simulink model "gm_HDL_pfc_gold_fi_og_vnl"  (R2024b)
settings: Solver=FixedStepDiscrete  StartTime=0.0  StopTime=.2  RelTol=1e-3
InitFcn:
  | fidelity_pfc_vals;
  | nbits=(2^12)-2;
  | load('C:\Users\Angel\Desktop\hil\pfc3ph\matlab\sim\sschdl\pfc_desktop\stateSpaceParameters.mat');
undefined symbols (not defined in the file or in its folder): a, b, c, DiscIntNeverNeededParam, fsw, Gs, s, stateSpaceParameters_1, t_ss, tsw
libraries: simulink x47, hdlmdlgenlib x24, hdlsllib x10, mcbcontrolslib x5, dspsrcs4 x3, slpidlib x2, hdlssclib x2, spsSVPWMGenerator2LevelLib x1, spsPLL3phLib x1, fillib x1
(part 5 of 5)

== system gm_HDL_pfc_gold_fi_og_vnl/simscape_system/simscape_system/HDL Subsystem/Sparse Matrix-Vector Product3/hNNewMatrixD_shared/Serializer_Subnetwork ==
  in0 : Inport  OutDataTypeStr=fixdt(1, 25, 19)  PortDimensions=[140]  SampleTime=1.38600138600139e-08
  in1 : Inport  Port=2  OutDataTypeStr=fixdt(0, 5, 0)  SampleTime=1.38600138600139e-08
  ratechange_splitcomp : Demux  Outputs=20
  splitcomp_multiport : MultiPortSwitch  DataPortOrder=Zero-based contiguous  Inputs=20  DiagnosticForDefault=None  zeroidx=on  OutDataTypeStr=fixdt(1, 25, 19)  SampleTime=1.38600138600139e-08  SaturateOnIntegerOverflow=off  InputSameDT=off
  out0 : Outport  OutDataTypeStr=fixdt(1, 25, 19)  PortDimensions=[7]  SampleTime=1.38600138600139e-08
  wires:
  splitcomp_multiport/1 -> out0/1
  ratechange_splitcomp/20 -> splitcomp_multiport/21
  ratechange_splitcomp/19 -> splitcomp_multiport/20
  ratechange_splitcomp/14 -> splitcomp_multiport/15
  ratechange_splitcomp/16 -> splitcomp_multiport/17
  ratechange_splitcomp/13 -> splitcomp_multiport/14
  ratechange_splitcomp/15 -> splitcomp_multiport/16
  ratechange_splitcomp/12 -> splitcomp_multiport/13
  ratechange_splitcomp/10 -> splitcomp_multiport/11
  ratechange_splitcomp/17 -> splitcomp_multiport/18
  ratechange_splitcomp/7 -> splitcomp_multiport/8
  ratechange_splitcomp/9 -> splitcomp_multiport/10
  ratechange_splitcomp/6 -> splitcomp_multiport/7
  ratechange_splitcomp/8 -> splitcomp_multiport/9
  ratechange_splitcomp/4 -> splitcomp_multiport/5
  in1/1 -> splitcomp_multiport/1
  ratechange_splitcomp/1 -> splitcomp_multiport/2
  in0/1 -> ratechange_splitcomp/1
  ratechange_splitcomp/2 -> splitcomp_multiport/3
  ratechange_splitcomp/3 -> splitcomp_multiport/4
  ratechange_splitcomp/5 -> splitcomp_multiport/6
  ratechange_splitcomp/11 -> splitcomp_multiport/12
  ratechange_splitcomp/18 -> splitcomp_multiport/19

== system gm_HDL_pfc_gold_fi_og_vnl/simscape_system/simscape_system/HDL Subsystem/Sparse Matrix-Vector Product3/hNNewMatrixD_shared/Serializer_Subnetwork1 ==
  in0 : Inport  OutDataTypeStr=fixdt(1, 25, 13)  PortDimensions=[140]  SampleTime=1.38600138600139e-08
  in1 : Inport  Port=2  OutDataTypeStr=fixdt(0, 5, 0)  SampleTime=1.38600138600139e-08
  ratechange_splitcomp : Demux  Outputs=20
  splitcomp_multiport : MultiPortSwitch  DataPortOrder=Zero-based contiguous  Inputs=20  DiagnosticForDefault=None  zeroidx=on  OutDataTypeStr=fixdt(1, 25, 13)  SampleTime=1.38600138600139e-08  SaturateOnIntegerOverflow=off  InputSameDT=off
  out0 : Outport  OutDataTypeStr=fixdt(1, 25, 13)  PortDimensions=[7]  SampleTime=1.38600138600139e-08
  wires:
  ratechange_splitcomp/16 -> splitcomp_multiport/17
  ratechange_splitcomp/18 -> splitcomp_multiport/19
  ratechange_splitcomp/20 -> splitcomp_multiport/21
  ratechange_splitcomp/14 -> splitcomp_multiport/15
  ratechange_splitcomp/13 -> splitcomp_multiport/14
  ratechange_splitcomp/12 -> splitcomp_multiport/13
  ratechange_splitcomp/11 -> splitcomp_multiport/12
  ratechange_splitcomp/10 -> splitcomp_multiport/11
  ratechange_splitcomp/9 -> splitcomp_multiport/10
  splitcomp_multiport/1 -> out0/1
  ratechange_splitcomp/7 -> splitcomp_multiport/8
  ratechange_splitcomp/3 -> splitcomp_multiport/4
  ratechange_splitcomp/4 -> splitcomp_multiport/5
  ratechange_splitcomp/5 -> splitcomp_multiport/6
  ratechange_splitcomp/1 -> splitcomp_multiport/2
  ratechange_splitcomp/15 -> splitcomp_multiport/16
  ratechange_splitcomp/17 -> splitcomp_multiport/18
  ratechange_splitcomp/19 -> splitcomp_multiport/20
  in1/1 -> splitcomp_multiport/1
  ratechange_splitcomp/2 -> splitcomp_multiport/3
  ratechange_splitcomp/6 -> splitcomp_multiport/7
  ratechange_splitcomp/8 -> splitcomp_multiport/9
  in0/1 -> ratechange_splitcomp/1

== system gm_HDL_pfc_gold_fi_og_vnl/simscape_system/simscape_system/HDL Subsystem/Sparse Matrix-Vector Product3/hNNewMatrixD_shared/counter ==
  globalSchedule : EnablePort  OutDataTypeStr=boolean
  ctr_0_19 : hdlsllib/Sources/HDL Counter  CountType=Count limited  CountInit=double(0)  CountStep=double(1)  CountMax=double(19)  CountFromType=Initial value  CountFrom=double(0)  CountResetPort=off  CountLoadPort=off  CountEnbPort=off  CountDirPort=off  CountHitOutputPort=off  CountDataType=Unsigned  CountWordLen=5  CountFracLen=0  CountSampTime=1.38600138600139e-08
  out0 : Outport  OutDataTypeStr=fixdt(0, 5, 0)  SampleTime=1.38600138600139e-08  InitialOutput=0
  wires:
  ctr_0_19/1 -> out0/1

== system gm_HDL_pfc_gold_fi_og_vnl/simscape_system/simscape_system/HDL Subsystem/Sparse Matrix-Vector Product3/hNNewMatrixD_shared/dot_product1_bypass ==
  in0 : Inport  OutDataTypeStr=fixdt(1, 50, 32)  SampleTime=1.38600138600139e-08
  in1 : Inport  Port=2  OutDataTypeStr=boolean  SampleTime=1.38600138600139e-08
  dot_product1_enb : Switch  Criteria=u2 ~= 0  Threshold=double(0)  OutDataTypeStr=fixdt(1, 50, 32)  SampleTime=1.38600138600139e-08  SaturateOnIntegerOverflow=off  InputSameDT=off
  dot_product1_state : Delay  DelayLength=double(1)  InitialCondition=0  SampleTime=1.38600138600139e-08
  out0 : Outport  OutDataTypeStr=fixdt(1, 50, 32)  SampleTime=1.38600138600139e-08
  wires:
  dot_product1_state/1 -> dot_product1_enb/3
  in1/1 -> dot_product1_enb/2
  in0/1 -> dot_product1_enb/1
  dot_product1_enb/1 -> out0/1, dot_product1_state/1

== system gm_HDL_pfc_gold_fi_og_vnl/simscape_system/simscape_system/HDL Subsystem/Sparse Matrix-Vector Product3/hNNewMatrixD_shared/dot_product_7 ==
  in1 : Inport  OutDataTypeStr=fixdt(1, 25, 19)  PortDimensions=[7]  SampleTime=1.38600138600139e-08
  in2 : Inport  Port=2  OutDataTypeStr=fixdt(1, 25, 13)  PortDimensions=[7]  SampleTime=1.38600138600139e-08
  HwModeRegister : Delay  DelayLength=double(1)  InitialCondition=0  SampleTime=1.38600138600139e-08
  HwModeRegister1 : Delay  DelayLength=double(1)  InitialCondition=0  SampleTime=1.38600138600139e-08
  PipelineRegister : Delay  DelayLength=double(1)  InitialCondition=0  SampleTime=1.38600138600139e-08
  adder{,1..5} (6 alike) : Sum  OutDataTypeStr=fixdt(1, 50, 32)  SampleTime=1.38600138600139e-08
  mul_out1_6_wire : hdlmdlgenlib/Buffer
  multiplier : Product  Inputs=**  OutDataTypeStr=fixdt(1, 50, 32)  SampleTime=1.38600138600139e-08
  rd_0 : Delay  DelayLength=double(5)  InitialCondition=0  SampleTime=1.38600138600139e-08
  sum_stage3_1_wire : hdlmdlgenlib/Buffer
  t : Demux  Outputs=7
  out1 : Outport  OutDataTypeStr=fixdt(1, 50, 32)  SampleTime=1.38600138600139e-08
  wires:
  sum_stage3_1_wire/1 -> out1/1
  adder4/1 -> adder5/2
  adder5/1 -> sum_stage3_1_wire/1
  adder3/1 -> adder5/1
  mul_out1_6_wire/1 -> adder4/2
  adder2/1 -> adder4/1
  adder1/1 -> adder3/2
  adder/1 -> adder3/1
  t/3 -> adder1/1
  t/5 -> adder2/1
  t/7 -> mul_out1_6_wire/1
  t/2 -> adder/2
  t/4 -> adder1/2
  t/6 -> adder2/2
  HwModeRegister1/1 -> multiplier/2
  rd_0/1 -> HwModeRegister/1
  PipelineRegister/1 -> t/1
  t/1 -> adder/1
  in1/1 -> rd_0/1
  in2/1 -> HwModeRegister1/1
  HwModeRegister/1 -> multiplier/1
  multiplier/1 -> PipelineRegister/1

== system gm_HDL_pfc_gold_fi_og_vnl/simscape_system/simscape_system/HDL Subsystem/Sparse Matrix-Vector Product3/hNNewMatrixD_shared/tappedDelay ==
  in0 : Inport  OutDataTypeStr=fixdt(1, 50, 32)  SampleTime=1.38600138600139e-08
  globalSchedule : EnablePort  OutDataTypeStr=boolean
  StateControl : StateControl  StateControl=Synchronous
  tappedDelay : simulink/Discrete/Tapped Delay  vinit=0  samptime=-1  NumDelays=double(19)  DelayOrder=Oldest  includeCurrent=off
  out0 : Outport  OutDataTypeStr=fixdt(1, 50, 32)  PortDimensions=[19]  SampleTime=1.38600138600139e-08  InitialOutput=0
  wires:
  tappedDelay/1 -> out0/1
  in0/1 -> tappedDelay/1
